simulink model "sim_quartercar"  (R2023b)
settings: Solver=FixedStepAuto  StartTime=0.0  StopTime=10.0  FixedStep=0.001  RelTol=1e-3
values from neighbouring files (symbols this model uses):
  A = [ 0 1 0 0;            [-ks -bs ks bs]/ms;            0 0 0 1;            [ks bs -ks-kt -bs]/mu]    [caller_sims.m]    (also in example_actsusp_bd.m = [ 0 1 0 0; [-ks -bs ks bs]/mb ;        0 0 0 1; [ks bs -ks-k; example_lpv_output_feedback_claude.m = [ 0   1; example_lpv_state_feedback_claude.m = [ 0   1; model_activevibrationisolator.m = [0, 0;      1, 0])
  B = [ 0 0; 0 1e3/ms; 0 0; [kt -1e3]/mu]    [caller_sims.m]    (also in example_actsusp_bd.m = [ 0 0; 0 1e3/mb ; 0 0 ; [kt -1e3]/mw]; example_lpv_output_feedback_claude.m = [0; 1]; example_lpv_state_feedback_claude.m = [0; 1]; model_activevibrationisolator.m = [1/M;      0])
  bs = 800    [caller_sims.m]    (also in example_actsusp_bd.m = 1000; model_quatercar_bd.m = 1000; model_rajavani_actsus_modifiedhinf.m = 1000; run.m = 1000)
  ks = 15000    [caller_sims.m]    (also in example_actsusp_bd.m = 16000; model_quatercar_bd.m = 16000; model_rajavani_actsus_modifiedhinf.m = 16000; run.m = 16000)
  kt = 120000    [caller_sims.m]    (also in example_actsusp_bd.m = 190000; model_quatercar_bd.m = 190000; model_rajavani_actsus_modifiedhinf.m = 160000; run.m = 160000)
  mb = 300    [example_actsusp_bd.m]    (also in model_quatercar_bd.m; run_updated.m = 250; sim_quartercar_hinf.m)
  mw = 60    [example_actsusp_bd.m]    (also in model_quatercar_bd.m; run_updated.m = 35; sim_quartercar_hinf.m)
libraries: slpidlib x1
settings Model: Creator=yusufcagriogut  LastModifiedBy=yusufcagriogut

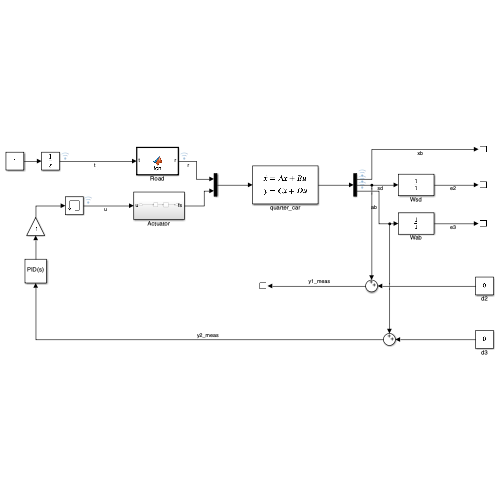
[thumbnail: Simulink's stored preview of the top-level diagram]
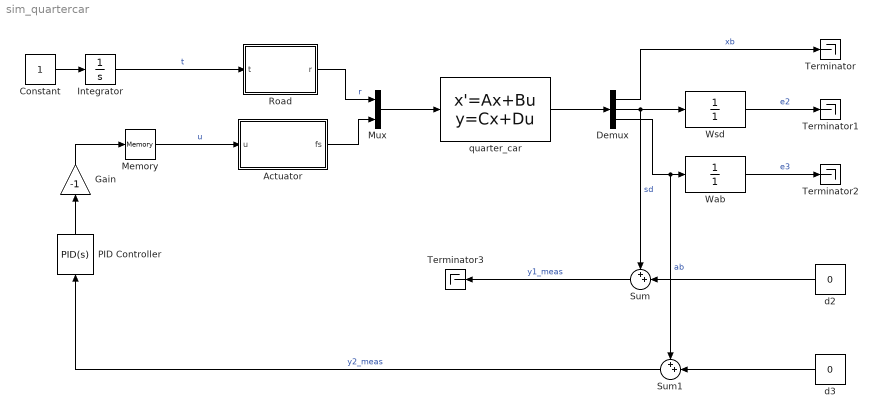
== system sim_quartercar ==
  Actuator : Subsystem
  Constant : Constant
  Demux : Demux  Outputs=3
  Gain : Gain  Gain=-1
  Integrator : Integrator
  Memory : Memory
  Mux : Mux  Inputs=2
  PID Controller : slpidlib/PID Controller  Controller=PID  Form=Parallel  TimeDomain=Continuous-time  UseExternalTs=off  SampleTime=-1  IntegratorMethod=Forward Euler  FilterMethod=Forward Euler  ControllerParametersSource=internal  P=0.1  I=1  UseKiTs=off  D=0  N=100  UseFilter=on  TunerSelectOption=Transfer Function Based (PID Tuner App)  InitialConditionSource=internal  InitialConditionForIntegrator=0  InitialConditionForFilter=0  DifferentiatorICPrevScaledInput=0  ExternalReset=none  TrackingMode=off  Kt=1  LimitOutput=off  SatLimitsSource=internal  UpperSaturationLimit=inf  LowerSaturationLimit=-inf  LinearizeAsGain=on  AntiWindupMode=none  Kb=1  LimitIntegrator=off  UpperIntegratorSaturationLimit=inf  LowerIntegratorSaturationLimit=-inf  POutMin=[]  POutMax=[]  IOutMin=[]  IOutMax=[]  DOutMin=[]  DOutMax=[]  NOutMin=[]  NOutMax=[]  SumOutMin=[]  SumOutMax=[]  SaturationOutMin=[]  SaturationOutMax=[]  PParamMin=[]  PParamMax=[]  IParamMin=[]  IParamMax=[]  DParamMin=[]  DParamMax=[]  NParamMin=[]  NParamMax=[]  KbParamMin=[]  KbParamMax=[]  KtParamMin=[]  KtParamMax=[]  KbOutMin=[]  KbOutMax=[]  KtOutMin=[]  KtOutMax=[]  IntegratorOutMin=[]  IntegratorOutMax=[]  FilterOutMin=[]  FilterOutMax=[]  SumI1OutMin=[]  SumI1OutMax=[]  SumI2OutMin=[]  SumI2OutMax=[]  SumI3OutMin=[]  SumI3OutMax=[]  SumI4OutMin=[]  SumI4OutMax=[]  SumDOutMin=[]  SumDOutMax=[]  DifferentiatorOutMin=[]  DifferentiatorOutMax=[]  FilterDiffOutCoefMin=[]  FilterDiffOutCoefMax=[]  ReciprocalOutMin=[]  ReciprocalOutMax=[]  SumDenOutMin=[]  SumDenOutMax=[]  SumNumOutMin=[]  SumNumOutMax=[]  DivideOutMin=[]  DivideOutMax=[]  UdiffTsProdOutMin=[]  UdiffTsProdOutMax=[]  NTsProdOutMin=[]  NTsProdOutMax=[]  UintegralTsProdOutMin=[]  UintegralTsProdOutMax=[]  UngainTsProdOutMin=[]  UngainTsProdOutMax=[]  ClampingZeroOutDataTypeStr=Inherit: Inherit via back propagation  ClampingZeroOutMin=[]  ClampingZeroOutMax=[]  FilterDenConstantOutDataTypeStr=Inherit: Inherit via back propagation  FilterDenConstantOutMin=[]  FilterDenConstantOutMax=[]  PCopyOutDataTypeStr=Inherit: Inherit via back propagation  PCopyOutMin=[]  PCopyOutMax=[]  NCopyOutDataTypeStr=Inherit: Inherit via back propagation  NCopyOutMin=[]  NCopyOutMax=[]  IntegratorContinuousStateAttributes=''  IntegratorStateMustResolveToSignalObject=off  IntegratorRTWStateStorageClass=Auto  FilterContinuousStateAttributes=''  FilterStateMustResolveToSignalObject=off  FilterRTWStateStorageClass=Auto  ParallelPVariant=InternalParameters  IdealPVariant=Disabled  IVariant=InternalParameters  DVariant=InternalParameters  IntegratorVariant=Continuous  SatVariant=Disabled  AWVariant=Passthrough  PCopyVariant=Disabled  TRVariant=Disabled  FdbkBlocksVariant=Forward  IdealPFdbkVariant=Disabled  SatFdbkVariant=Disabled  DerivativeFilterVariant=ContFilter  NVariant=InternalParameters  NCopyVariant=Disabled  FilterICVariant=InternalICsFilter  IntegratorICVariant=InternalICs  ExternalResetVariant=Disabled  TRSumVariant=Passthrough  SumFdbkVariant=Disabled  SumVariant=Sum_PID  TsampFilterVariant=InternalTs  TsampNgainVariant=Passthrough  TsampIntegralVariant=Disabled_SignalSpec  ExternalSaturationOutDataTypeStr=Inherit: Same as second input
  Road : MATLAB Function  TreatAsAtomicUnit=on
  Sum : Sum  Inputs=++|
  Sum1 : Sum  Inputs=++|
  Terminator{,1..3} (4 alike) : Terminator
  Wab : TransferFcn  Denominator=[1]
  Wsd : TransferFcn  Denominator=[1]
  d2 : Constant  Value=0
  d3 : Constant  Value=0
  quarter_car : StateSpace  A=[ 0 1 0 0; [-ks -bs ks bs]/mb ; 0 0 0 1; [ks bs -ks-kt -bs]/mw];  B=[ 0 0; 0 1e3/mb ; 0 0 ; [kt -1e3]/mw];  C=[1 0 0 0; 1 0 -1 0; A(2,:)];  D=[0 0; 0 0; B(2,:)];  InitialCondition=0
  wires:
  Road/1(r) -> Mux/1  "r"
  Mux/1 -> quarter_car/1
  quarter_car/1 -> Demux/1
  Demux/1 -> Terminator/1  "xb"
  Demux/2 -> Sum/1, Wsd/1  "sd"
  Demux/3 -> Wab/1, Sum1/1  "ab"
  Wsd/1 -> Terminator1/1  "e2"
  Wab/1 -> Terminator2/1  "e3"
  d2/1 -> Sum/2
  d3/1 -> Sum1/2
  Sum/1 -> Terminator3/1  "y1_meas"
  Sum1/1 -> PID Controller/1  "y2_meas"
  PID Controller/1 -> Gain/1
  Constant/1 -> Integrator/1
  Integrator/1 -> Road/1(t)  "t"
  Gain/1 -> Memory/1
  Memory/1 -> Actuator/1(u)  "u"
  Actuator/1(fs) -> Mux/2

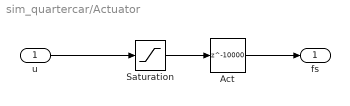
== system sim_quartercar/Actuator ==
  u : Inport
  Act : Delay  DelayLength=10000
  Saturation : Saturate  UpperLimit=100  LowerLimit=-100
  fs : Outport
  wires:
  Act/1 -> fs/1
  u/1 -> Saturation/1
  Saturation/1 -> Act/1

== matlab function sim_quartercar/Road ==
  data: t input; r output
function r = fcn(t)
t_start = 0.5; t_end = 0.7; t_diff = t_end - t_start;
if t>=t_start && t<=t_end
    % r = sind((t-t_start)*180/t_diff);
    r = 0.1;
else
    r = 0;
end
